simulink model "determination_PI"  (R2024a)
settings: Solver=VariableStepAuto  StartTime=0.0  StopTime=0.2  RelTol=1e-3
undefined symbols (not defined in the file): Co, f, J, Kphi, L, R, Rch
settings Model: Creator=mguerchon01  LastModifiedBy=magic

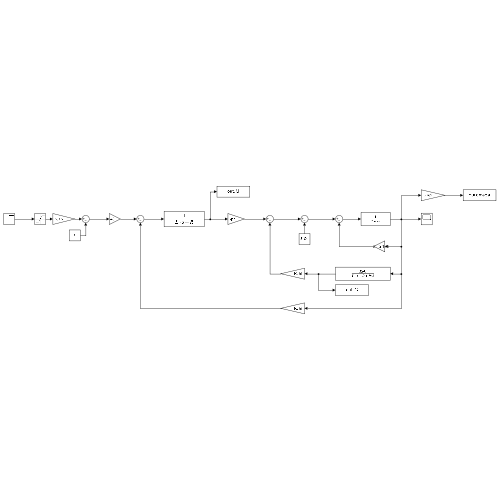
[thumbnail: Simulink's stored preview of the top-level diagram]
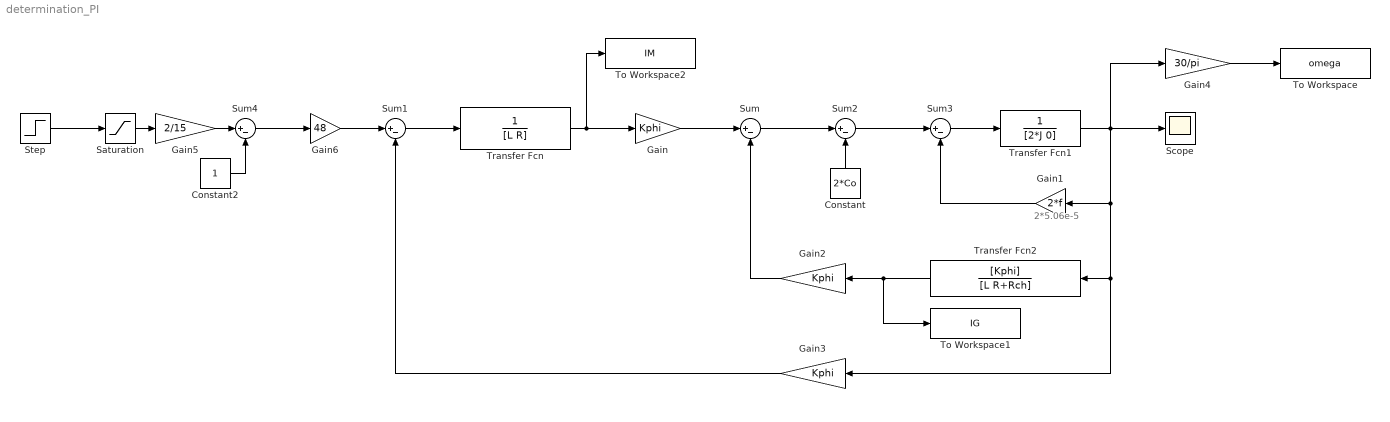
== system determination_PI ==
  note: 2*5.06e-5
  Constant : Constant  Value=2*Co
  Constant2 : Constant
  Gain : Gain  Gain=Kphi
  Gain1 : Gain  Gain=2*f
  Gain2 : Gain  Gain=Kphi
  Gain3 : Gain  Gain=Kphi
  Gain4 : Gain  Gain=30/pi
  Gain5 : Gain  Gain=2/15
  Gain6 : Gain  Gain=48
  Saturation : Saturate  UpperLimit=14.9  LowerLimit=0.1
  Scope : Scope
  Step : Step  After=15  SampleTime=0
  Sum{,1..4} (5 alike) : Sum  Inputs=|+-
  To Workspace : ToWorkspace  VariableName=omega  SaveFormat=Timeseries  SampleTime=-1
  To Workspace1 : ToWorkspace  VariableName=IG  SaveFormat=Timeseries  SampleTime=-1
  To Workspace2 : ToWorkspace  VariableName=IM  SaveFormat=Timeseries  SampleTime=-1
  Transfer Fcn : TransferFcn  Denominator=[L R]
  Transfer Fcn1 : TransferFcn  Denominator=[2*J 0]
  Transfer Fcn2 : TransferFcn  Numerator=[Kphi]  Denominator=[L R+Rch]
  wires:
  Transfer Fcn/1 -> To Workspace2/1, Gain/1
  Sum1/1 -> Transfer Fcn/1
  Gain/1 -> Sum/1
  Constant/1 -> Sum2/2
  Sum2/1 -> Sum3/1
  Sum/1 -> Sum2/1
  Sum3/1 -> Transfer Fcn1/1
  Transfer Fcn1/1 -> Gain4/1, Scope/1, Gain3/1, Transfer Fcn2/1, Gain1/1
  Gain1/1 -> Sum3/2
  Transfer Fcn2/1 -> To Workspace1/1, Gain2/1
  Gain2/1 -> Sum/2
  Gain3/1 -> Sum1/2
  Gain4/1 -> To Workspace/1
  Gain6/1 -> Sum1/1
  Saturation/1 -> Gain5/1
  Gain5/1 -> Sum4/1
  Constant2/1 -> Sum4/2
  Sum4/1 -> Gain6/1
  Step/1 -> Saturation/1
